simulink model "ddc_bpm_476_066_bak5"  (Simulink 7.8)
settings: Solver=ode45  StartTime=0.0  StopTime=2.56e-3  RelTol=1e-3
undefined symbols (not defined in the file): dt_sim, frev_476, Fs_adc, xlipgetpartsetting
libraries: xbsIndex_r4 x605, simulink x3
(part 2 of 6)

== system ddc_bpm_476_066_bak5/Channel1_fofb ==
  Mix_q_in : Inport
  Mix_i_in : Inport  Port=2
  Analysis : Subsystem
  Goto Tag Visibility3 : GotoTagVisibility  GotoTag=CIC_FOFB_Q_FPGA_OUT
  Goto Tag Visibility4 : GotoTagVisibility  GotoTag=CIC_FOFB_I_FPGA_OUT
  Goto Tag Visibility5 : GotoTagVisibility  GotoTag=CORDIC_FOFB_T_FPGA_OUT
  Goto Tag Visibility6 : GotoTagVisibility  GotoTag=CORDIC_FOFB_R_FPGA_OUT
  Register4 : xbsIndex_r4/Register  init=0  rst=off  en=on  dbl_ovrd=off  block_type=register
  Register5 : xbsIndex_r4/Register  init=0  rst=off  en=on  dbl_ovrd=off  block_type=register
  Register6 : xbsIndex_r4/Register  init=0  rst=off  en=off  dbl_ovrd=off  block_type=register
  Reinterpret2 : xbsIndex_r4/Reinterpret  force_arith_type=off  arith_type=Unsigned  force_bin_pt=off  bin_pt=18  block_type=reinterpret
  Reinterpret3 : xbsIndex_r4/Reinterpret  force_arith_type=off  arith_type=Unsigned  force_bin_pt=off  bin_pt=19  block_type=reinterpret
  Terminator{1,5,8..9} (4 alike) : Terminator
  cic_fofb : Subsystem
  cic_fofb_ch1_i_o : xbsIndex_r4/Gateway Out  inherit_from_input=on  hdl_port=on  timing_constraint=Data Rate  locs_specified=off  LOCs={}  UseAsDAC=off  DACChannel='1'  block_type=gatewayout
      settings: infoedit="Gateway out block.  Converts Xilinx fixed-point or floating-point type inputs into ouputs of type Simulink integer, single, double, or fixed point.<br><br>Hardware notes:  In hardware these blocks become top level output ports or are discarded, depending on how they are configured."
  cic_fofb_ch1_q_o : xbsIndex_r4/Gateway Out  inherit_from_input=on  hdl_port=on  timing_constraint=Data Rate  locs_specified=off  LOCs={}  UseAsDAC=off  DACChannel='1'  block_type=gatewayout
      settings: infoedit="Gateway out block.  Converts Xilinx fixed-point or floating-point type inputs into ouputs of type Simulink integer, single, double, or fixed point.<br><br>Hardware notes:  In hardware these blocks become top level output ports or are discarded, depending on how they are configured."
  fofb_amp_ch1_o : xbsIndex_r4/Gateway Out  inherit_from_input=on  hdl_port=on  timing_constraint=Data Rate  locs_specified=off  LOCs={}  UseAsDAC=off  DACChannel='1'  block_type=gatewayout
      settings: infoedit="Gateway out block.  Converts Xilinx fixed-point or floating-point type inputs into ouputs of type Simulink integer, single, double, or fixed point.<br><br>Hardware notes:  In hardware these blocks become top level output ports or are discarded, depending on how they are configured."
  rect2pol : xbsIndex_r4/CORDIC 5.0   functional_selection=Translate  architectural_configuration=Parallel  pipelining_mode=Maximum  data_format=SignedFraction  phase_format=Radians  input_width=24  output_width=24  round_mode=Nearest_Even  iterations=0  precision=0  compensation_scaling=BRAM  coarse_rotation=on  aclken=off  aresetn=off  out_tready=off  cartesian_has_tuser=off  cartesian_has_tlast=off  cartesian_tuser_width=1  phase_has_tuser=off  phase_has_tlast=off  phase_tuser_width=1  out_tlast_behv=Null  flow_control=NonBlocking  optimize_goal=Resources  trim_axipin_name=on  ip_name=CORDIC  ip_version=5.0  dsptool_ready=true  ipcore_usecache=true  ipcore_useipmodelcache=true  wrapper_available=true  port_translation_map={ 'aclken' => 'en', 'aresetn' => 'rst' }  block_type=cordic_v5_0
      settings: infoedit=CORDIC 5.0
  Amp_F : Outport
  Phase_F : Outport  Port=2
  Valid_F : Outport  Port=3
  tag scope: CIC_FOFB_I_FPGA_OUT=scoped, CIC_FOFB_Q_FPGA_OUT=scoped, CORDIC_FOFB_R_FPGA_OUT=scoped, CORDIC_FOFB_T_FPGA_OUT=scoped
  wires:
  cic_fofb/3(I_out) -> cic_fofb_ch1_i_o/1, [CIC_FOFB_I_FPGA_OUT], rect2pol/3
  cic_fofb/1(Q_out) -> [CIC_FOFB_Q_FPGA_OUT], cic_fofb_ch1_q_o/1, rect2pol/2
  cic_fofb/2(Q_valid) -> Terminator1/1
  rect2pol/1 -> Register4/2, Register5/2, Register6/1
  rect2pol/2 -> Reinterpret2/1
  rect2pol/3 -> Reinterpret3/1
  Register4/1 -> Phase_F/1, [CORDIC_FOFB_T_FPGA_OUT]
  Register5/1 -> Amp_F/1, [CORDIC_FOFB_R_FPGA_OUT], fofb_amp_ch1_o/1
  Register6/1 -> Valid_F/1
  Reinterpret2/1 -> Register4/1
  Reinterpret3/1 -> Register5/1
  fofb_amp_ch1_o/1 -> Terminator5/1
  cic_fofb_ch1_q_o/1 -> Terminator9/1
  cic_fofb_ch1_i_o/1 -> Terminator8/1
  Mix_q_in/1 -> cic_fofb/1(Q_in)
  Mix_i_in/1 -> cic_fofb/2(I_in)
  cic_fofb/4(I_valid) -> rect2pol/1

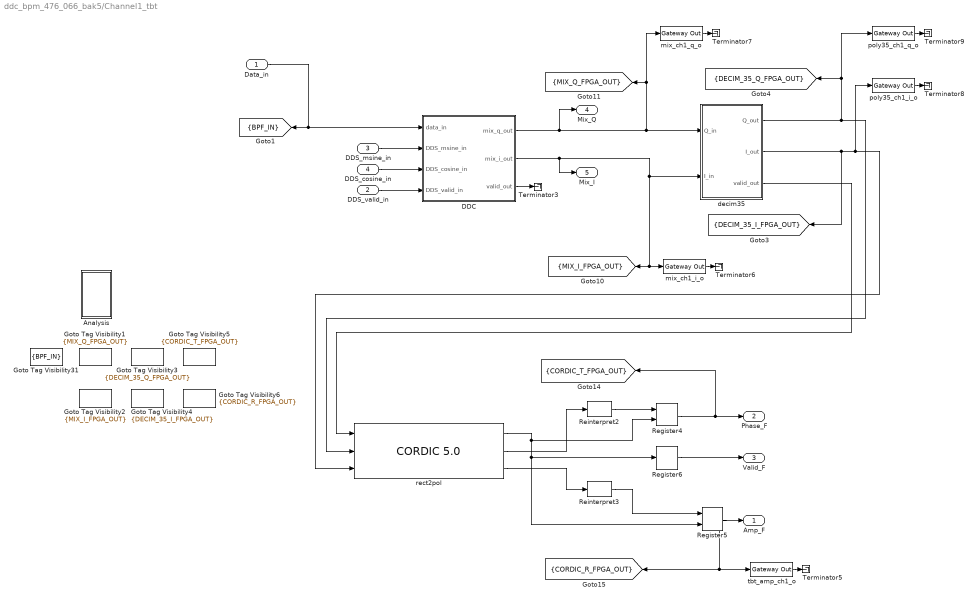
== system ddc_bpm_476_066_bak5/Channel1_tbt ==
  Data_in : Inport
  DDS_valid_in : Inport  Port=2
  DDS_msine_in : Inport  Port=3
  DDS_cosine_in : Inport  Port=4
  Analysis : Subsystem
  DDC : Subsystem
  Goto Tag Visibility1 : GotoTagVisibility  GotoTag=MIX_Q_FPGA_OUT
  Goto Tag Visibility2 : GotoTagVisibility  GotoTag=MIX_I_FPGA_OUT
  Goto Tag Visibility3 : GotoTagVisibility  GotoTag=DECIM_35_Q_FPGA_OUT
  Goto Tag Visibility31 : GotoTagVisibility  GotoTag=BPF_IN
  Goto Tag Visibility4 : GotoTagVisibility  GotoTag=DECIM_35_I_FPGA_OUT
  Goto Tag Visibility5 : GotoTagVisibility  GotoTag=CORDIC_T_FPGA_OUT
  Goto Tag Visibility6 : GotoTagVisibility  GotoTag=CORDIC_R_FPGA_OUT
  Register4 : xbsIndex_r4/Register  init=0  rst=off  en=on  dbl_ovrd=off  block_type=register
  Register5 : xbsIndex_r4/Register  init=0  rst=off  en=on  dbl_ovrd=off  block_type=register
  Register6 : xbsIndex_r4/Register  init=0  rst=off  en=off  dbl_ovrd=off  block_type=register
  Reinterpret2 : xbsIndex_r4/Reinterpret  force_arith_type=off  arith_type=Unsigned  force_bin_pt=off  bin_pt=18  block_type=reinterpret
  Reinterpret3 : xbsIndex_r4/Reinterpret  force_arith_type=off  arith_type=Unsigned  force_bin_pt=off  bin_pt=19  block_type=reinterpret
  Terminator{3,5..9} (6 alike) : Terminator
  decim35 : Subsystem
  mix_ch1_i_o : xbsIndex_r4/Gateway Out  inherit_from_input=on  hdl_port=on  timing_constraint=Data Rate  locs_specified=off  LOCs={}  UseAsDAC=off  DACChannel='1'  block_type=gatewayout
      settings: infoedit="Gateway out block.  Converts Xilinx fixed-point or floating-point type inputs into ouputs of type Simulink integer, single, double, or fixed point.<br><br>Hardware notes:  In hardware these blocks become top level output ports or are discarded, depending on how they are configured."
  mix_ch1_q_o : xbsIndex_r4/Gateway Out  inherit_from_input=on  hdl_port=on  timing_constraint=Data Rate  locs_specified=off  LOCs={}  UseAsDAC=off  DACChannel='1'  block_type=gatewayout
      settings: infoedit="Gateway out block.  Converts Xilinx fixed-point or floating-point type inputs into ouputs of type Simulink integer, single, double, or fixed point.<br><br>Hardware notes:  In hardware these blocks become top level output ports or are discarded, depending on how they are configured."
  poly35_ch1_i_o : xbsIndex_r4/Gateway Out  inherit_from_input=on  hdl_port=on  timing_constraint=Data Rate  locs_specified=off  LOCs={}  UseAsDAC=off  DACChannel='1'  block_type=gatewayout
      settings: infoedit="Gateway out block.  Converts Xilinx fixed-point or floating-point type inputs into ouputs of type Simulink integer, single, double, or fixed point.<br><br>Hardware notes:  In hardware these blocks become top level output ports or are discarded, depending on how they are configured."
  poly35_ch1_q_o : xbsIndex_r4/Gateway Out  inherit_from_input=on  hdl_port=on  timing_constraint=Data Rate  locs_specified=off  LOCs={}  UseAsDAC=off  DACChannel='1'  block_type=gatewayout
      settings: infoedit="Gateway out block.  Converts Xilinx fixed-point or floating-point type inputs into ouputs of type Simulink integer, single, double, or fixed point.<br><br>Hardware notes:  In hardware these blocks become top level output ports or are discarded, depending on how they are configured."
  rect2pol : xbsIndex_r4/CORDIC 5.0   functional_selection=Translate  architectural_configuration=Parallel  pipelining_mode=Maximum  data_format=SignedFraction  phase_format=Radians  input_width=24  output_width=24  round_mode=Nearest_Even  iterations=0  precision=0  compensation_scaling=BRAM  coarse_rotation=on  aclken=off  aresetn=off  out_tready=off  cartesian_has_tuser=off  cartesian_has_tlast=off  cartesian_tuser_width=1  phase_has_tuser=off  phase_has_tlast=off  phase_tuser_width=1  out_tlast_behv=Null  flow_control=NonBlocking  optimize_goal=Resources  trim_axipin_name=on  ip_name=CORDIC  ip_version=5.0  dsptool_ready=true  ipcore_usecache=true  ipcore_useipmodelcache=true  wrapper_available=true  port_translation_map={ 'aclken' => 'en', 'aresetn' => 'rst' }  block_type=cordic_v5_0
      settings: infoedit=CORDIC 5.0
  tbt_amp_ch1_o : xbsIndex_r4/Gateway Out  inherit_from_input=on  hdl_port=on  timing_constraint=Data Rate  locs_specified=off  LOCs={}  UseAsDAC=off  DACChannel='1'  block_type=gatewayout
      settings: infoedit="Gateway out block.  Converts Xilinx fixed-point or floating-point type inputs into ouputs of type Simulink integer, single, double, or fixed point.<br><br>Hardware notes:  In hardware these blocks become top level output ports or are discarded, depending on how they are configured."
  Amp_F : Outport
  Phase_F : Outport  Port=2
  Valid_F : Outport  Port=3
  Mix_Q : Outport  Port=4
  Mix_I : Outport  Port=5
  tag scope: BPF_IN=scoped, CORDIC_R_FPGA_OUT=scoped, CORDIC_T_FPGA_OUT=scoped, DECIM_35_I_FPGA_OUT=scoped, DECIM_35_Q_FPGA_OUT=scoped, MIX_I_FPGA_OUT=scoped, MIX_Q_FPGA_OUT=scoped
  wires:
  Data_in/1 -> [BPF_IN], DDC/1(data_in)
  DDC/2(mix_i_out) -> [MIX_I_FPGA_OUT], mix_ch1_i_o/1, decim35/2(I_in), Mix_I/1
  DDC/3(valid_out) -> Terminator3/1
  DDC/1(mix_q_out) -> [MIX_Q_FPGA_OUT], mix_ch1_q_o/1, decim35/1(Q_in), Mix_Q/1
  decim35/2(I_out) -> [DECIM_35_I_FPGA_OUT], poly35_ch1_i_o/1, rect2pol/3
  decim35/1(Q_out) -> [DECIM_35_Q_FPGA_OUT], poly35_ch1_q_o/1, rect2pol/2
  decim35/3(valid_out) -> rect2pol/1
  rect2pol/1 -> Register4/2, Register5/2, Register6/1
  rect2pol/2 -> Reinterpret2/1
  rect2pol/3 -> Reinterpret3/1
  Register4/1 -> Phase_F/1, [CORDIC_T_FPGA_OUT]
  Register5/1 -> Amp_F/1, [CORDIC_R_FPGA_OUT], tbt_amp_ch1_o/1
  Register6/1 -> Valid_F/1
  Reinterpret2/1 -> Register4/1
  Reinterpret3/1 -> Register5/1
  tbt_amp_ch1_o/1 -> Terminator5/1
  mix_ch1_i_o/1 -> Terminator6/1
  mix_ch1_q_o/1 -> Terminator7/1
  poly35_ch1_q_o/1 -> Terminator9/1
  poly35_ch1_i_o/1 -> Terminator8/1
  DDS_valid_in/1 -> DDC/4(DDS_valid_in)
  DDS_msine_in/1 -> DDC/2(DDS_msine_in)
  DDS_cosine_in/1 -> DDC/3(DDS_cosine_in)

== system ddc_bpm_476_066_bak5/Channel2_fofb ==
  Mix_q_in : Inport
  Mix_i_in : Inport  Port=2
  Analysis : Subsystem
  Goto Tag Visibility3 : GotoTagVisibility  GotoTag=CIC_FOFB_Q_FPGA_OUT
  Goto Tag Visibility4 : GotoTagVisibility  GotoTag=CIC_FOFB_I_FPGA_OUT
  Goto Tag Visibility5 : GotoTagVisibility  GotoTag=CORDIC_FOFB_T_FPGA_OUT
  Goto Tag Visibility6 : GotoTagVisibility  GotoTag=CORDIC_FOFB_R_FPGA_OUT
  Register4 : xbsIndex_r4/Register  init=0  rst=off  en=on  dbl_ovrd=off  block_type=register
  Register5 : xbsIndex_r4/Register  init=0  rst=off  en=on  dbl_ovrd=off  block_type=register
  Register6 : xbsIndex_r4/Register  init=0  rst=off  en=off  dbl_ovrd=off  block_type=register
  Reinterpret2 : xbsIndex_r4/Reinterpret  force_arith_type=off  arith_type=Unsigned  force_bin_pt=off  bin_pt=18  block_type=reinterpret
  Reinterpret3 : xbsIndex_r4/Reinterpret  force_arith_type=off  arith_type=Unsigned  force_bin_pt=off  bin_pt=19  block_type=reinterpret
  Terminator{1,5,8..9} (4 alike) : Terminator
  cic_fofb : Subsystem
  cic_fofb_ch2_i_o : xbsIndex_r4/Gateway Out  inherit_from_input=on  hdl_port=on  timing_constraint=Data Rate  locs_specified=off  LOCs={}  UseAsDAC=off  DACChannel='1'  block_type=gatewayout
      settings: infoedit="Gateway out block.  Converts Xilinx fixed-point or floating-point type inputs into ouputs of type Simulink integer, single, double, or fixed point.<br><br>Hardware notes:  In hardware these blocks become top level output ports or are discarded, depending on how they are configured."
  cic_fofb_ch2_q_o : xbsIndex_r4/Gateway Out  inherit_from_input=on  hdl_port=on  timing_constraint=Data Rate  locs_specified=off  LOCs={}  UseAsDAC=off  DACChannel='1'  block_type=gatewayout
      settings: infoedit="Gateway out block.  Converts Xilinx fixed-point or floating-point type inputs into ouputs of type Simulink integer, single, double, or fixed point.<br><br>Hardware notes:  In hardware these blocks become top level output ports or are discarded, depending on how they are configured."
  fofb_amp_ch2_o : xbsIndex_r4/Gateway Out  inherit_from_input=on  hdl_port=on  timing_constraint=Data Rate  locs_specified=off  LOCs={}  UseAsDAC=off  DACChannel='1'  block_type=gatewayout
      settings: infoedit="Gateway out block.  Converts Xilinx fixed-point or floating-point type inputs into ouputs of type Simulink integer, single, double, or fixed point.<br><br>Hardware notes:  In hardware these blocks become top level output ports or are discarded, depending on how they are configured."
  rect2pol : xbsIndex_r4/CORDIC 5.0   functional_selection=Translate  architectural_configuration=Parallel  pipelining_mode=Maximum  data_format=SignedFraction  phase_format=Radians  input_width=24  output_width=24  round_mode=Nearest_Even  iterations=0  precision=0  compensation_scaling=BRAM  coarse_rotation=on  aclken=off  aresetn=off  out_tready=off  cartesian_has_tuser=off  cartesian_has_tlast=off  cartesian_tuser_width=1  phase_has_tuser=off  phase_has_tlast=off  phase_tuser_width=1  out_tlast_behv=Null  flow_control=NonBlocking  optimize_goal=Resources  trim_axipin_name=on  ip_name=CORDIC  ip_version=5.0  dsptool_ready=true  ipcore_usecache=true  ipcore_useipmodelcache=true  wrapper_available=true  port_translation_map={ 'aclken' => 'en', 'aresetn' => 'rst' }  block_type=cordic_v5_0
      settings: infoedit=CORDIC 5.0
  Amp_F : Outport
  Phase_F : Outport  Port=2
  Valid_F : Outport  Port=3
  tag scope: CIC_FOFB_I_FPGA_OUT=scoped, CIC_FOFB_Q_FPGA_OUT=scoped, CORDIC_FOFB_R_FPGA_OUT=scoped, CORDIC_FOFB_T_FPGA_OUT=scoped
  wires:
  cic_fofb/3(I_out) -> cic_fofb_ch2_i_o/1, [CIC_FOFB_I_FPGA_OUT], rect2pol/3
  cic_fofb/1(Q_out) -> [CIC_FOFB_Q_FPGA_OUT], cic_fofb_ch2_q_o/1, rect2pol/2
  cic_fofb/2(Q_valid) -> Terminator1/1
  rect2pol/1 -> Register4/2, Register5/2, Register6/1
  rect2pol/2 -> Reinterpret2/1
  rect2pol/3 -> Reinterpret3/1
  Register4/1 -> Phase_F/1, [CORDIC_FOFB_T_FPGA_OUT]
  Register5/1 -> Amp_F/1, [CORDIC_FOFB_R_FPGA_OUT], fofb_amp_ch2_o/1
  Register6/1 -> Valid_F/1
  Reinterpret2/1 -> Register4/1
  Reinterpret3/1 -> Register5/1
  fofb_amp_ch2_o/1 -> Terminator5/1
  cic_fofb_ch2_q_o/1 -> Terminator9/1
  cic_fofb_ch2_i_o/1 -> Terminator8/1
  Mix_q_in/1 -> cic_fofb/1(Q_in)
  Mix_i_in/1 -> cic_fofb/2(I_in)
  cic_fofb/4(I_valid) -> rect2pol/1

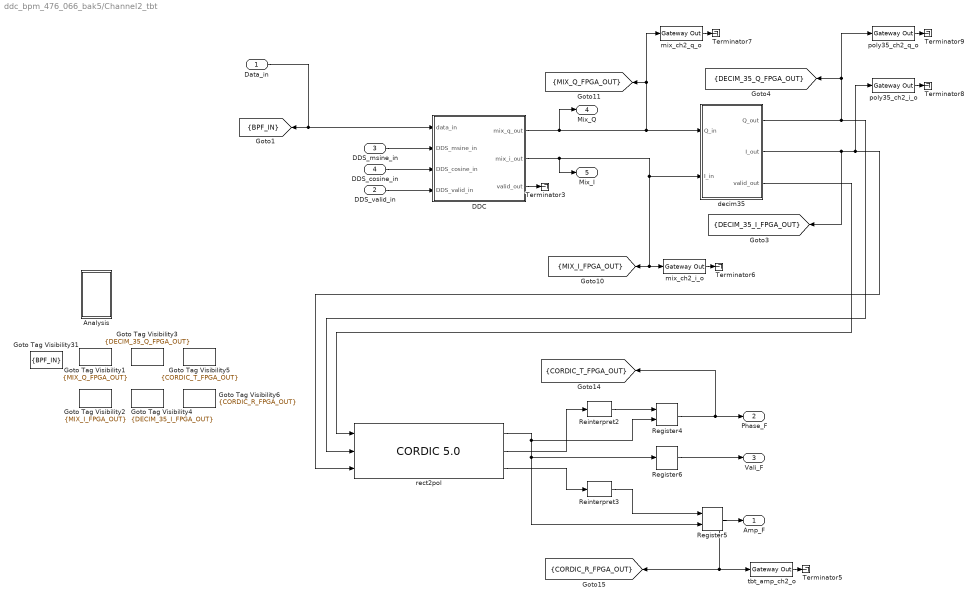
== system ddc_bpm_476_066_bak5/Channel2_tbt ==
  Data_in : Inport
  DDS_valid_in : Inport  Port=2
  DDS_msine_in : Inport  Port=3
  DDS_cosine_in : Inport  Port=4
  Analysis : Subsystem
  DDC : Subsystem
  Goto Tag Visibility1 : GotoTagVisibility  GotoTag=MIX_Q_FPGA_OUT
  Goto Tag Visibility2 : GotoTagVisibility  GotoTag=MIX_I_FPGA_OUT
  Goto Tag Visibility3 : GotoTagVisibility  GotoTag=DECIM_35_Q_FPGA_OUT
  Goto Tag Visibility31 : GotoTagVisibility  GotoTag=BPF_IN
  Goto Tag Visibility4 : GotoTagVisibility  GotoTag=DECIM_35_I_FPGA_OUT
  Goto Tag Visibility5 : GotoTagVisibility  GotoTag=CORDIC_T_FPGA_OUT
  Goto Tag Visibility6 : GotoTagVisibility  GotoTag=CORDIC_R_FPGA_OUT
  Register4 : xbsIndex_r4/Register  init=0  rst=off  en=on  dbl_ovrd=off  block_type=register
  Register5 : xbsIndex_r4/Register  init=0  rst=off  en=on  dbl_ovrd=off  block_type=register
  Register6 : xbsIndex_r4/Register  init=0  rst=off  en=off  dbl_ovrd=off  block_type=register
  Reinterpret2 : xbsIndex_r4/Reinterpret  force_arith_type=off  arith_type=Unsigned  force_bin_pt=off  bin_pt=18  block_type=reinterpret
  Reinterpret3 : xbsIndex_r4/Reinterpret  force_arith_type=off  arith_type=Unsigned  force_bin_pt=off  bin_pt=19  block_type=reinterpret
  Terminator{3,5..9} (6 alike) : Terminator
  decim35 : Subsystem
  mix_ch2_i_o : xbsIndex_r4/Gateway Out  inherit_from_input=on  hdl_port=on  timing_constraint=Data Rate  locs_specified=off  LOCs={}  UseAsDAC=off  DACChannel='1'  block_type=gatewayout
      settings: infoedit="Gateway out block.  Converts Xilinx fixed-point or floating-point type inputs into ouputs of type Simulink integer, single, double, or fixed point.<br><br>Hardware notes:  In hardware these blocks become top level output ports or are discarded, depending on how they are configured."
  mix_ch2_q_o : xbsIndex_r4/Gateway Out  inherit_from_input=on  hdl_port=on  timing_constraint=Data Rate  locs_specified=off  LOCs={}  UseAsDAC=off  DACChannel='1'  block_type=gatewayout
      settings: infoedit="Gateway out block.  Converts Xilinx fixed-point or floating-point type inputs into ouputs of type Simulink integer, single, double, or fixed point.<br><br>Hardware notes:  In hardware these blocks become top level output ports or are discarded, depending on how they are configured."
  poly35_ch2_i_o : xbsIndex_r4/Gateway Out  inherit_from_input=on  hdl_port=on  timing_constraint=Data Rate  locs_specified=off  LOCs={}  UseAsDAC=off  DACChannel='1'  block_type=gatewayout
      settings: infoedit="Gateway out block.  Converts Xilinx fixed-point or floating-point type inputs into ouputs of type Simulink integer, single, double, or fixed point.<br><br>Hardware notes:  In hardware these blocks become top level output ports or are discarded, depending on how they are configured."
  poly35_ch2_q_o : xbsIndex_r4/Gateway Out  inherit_from_input=on  hdl_port=on  timing_constraint=Data Rate  locs_specified=off  LOCs={}  UseAsDAC=off  DACChannel='1'  block_type=gatewayout
      settings: infoedit="Gateway out block.  Converts Xilinx fixed-point or floating-point type inputs into ouputs of type Simulink integer, single, double, or fixed point.<br><br>Hardware notes:  In hardware these blocks become top level output ports or are discarded, depending on how they are configured."
  rect2pol : xbsIndex_r4/CORDIC 5.0   functional_selection=Translate  architectural_configuration=Parallel  pipelining_mode=Maximum  data_format=SignedFraction  phase_format=Radians  input_width=24  output_width=24  round_mode=Nearest_Even  iterations=0  precision=0  compensation_scaling=BRAM  coarse_rotation=on  aclken=off  aresetn=off  out_tready=off  cartesian_has_tuser=off  cartesian_has_tlast=off  cartesian_tuser_width=1  phase_has_tuser=off  phase_has_tlast=off  phase_tuser_width=1  out_tlast_behv=Null  flow_control=NonBlocking  optimize_goal=Resources  trim_axipin_name=on  ip_name=CORDIC  ip_version=5.0  dsptool_ready=true  ipcore_usecache=true  ipcore_useipmodelcache=true  wrapper_available=true  port_translation_map={ 'aclken' => 'en', 'aresetn' => 'rst' }  block_type=cordic_v5_0
      settings: infoedit=CORDIC 5.0
  tbt_amp_ch2_o : xbsIndex_r4/Gateway Out  inherit_from_input=on  hdl_port=on  timing_constraint=Data Rate  locs_specified=off  LOCs={}  UseAsDAC=off  DACChannel='1'  block_type=gatewayout
      settings: infoedit="Gateway out block.  Converts Xilinx fixed-point or floating-point type inputs into ouputs of type Simulink integer, single, double, or fixed point.<br><br>Hardware notes:  In hardware these blocks become top level output ports or are discarded, depending on how they are configured."
  Amp_F : Outport
  Phase_F : Outport  Port=2
  Vali_F : Outport  Port=3
  Mix_Q : Outport  Port=4
  Mix_I : Outport  Port=5
  tag scope: BPF_IN=scoped, CORDIC_R_FPGA_OUT=scoped, CORDIC_T_FPGA_OUT=scoped, DECIM_35_I_FPGA_OUT=scoped, DECIM_35_Q_FPGA_OUT=scoped, MIX_I_FPGA_OUT=scoped, MIX_Q_FPGA_OUT=scoped
  wires:
  Data_in/1 -> [BPF_IN], DDC/1(data_in)
  DDC/2(mix_i_out) -> [MIX_I_FPGA_OUT], mix_ch2_i_o/1, decim35/2(I_in), Mix_I/1
  DDC/3(valid_out) -> Terminator3/1
  DDC/1(mix_q_out) -> [MIX_Q_FPGA_OUT], mix_ch2_q_o/1, decim35/1(Q_in), Mix_Q/1
  decim35/2(I_out) -> [DECIM_35_I_FPGA_OUT], poly35_ch2_i_o/1, rect2pol/3
  decim35/1(Q_out) -> [DECIM_35_Q_FPGA_OUT], poly35_ch2_q_o/1, rect2pol/2
  decim35/3(valid_out) -> rect2pol/1
  rect2pol/1 -> Register4/2, Register5/2, Register6/1
  rect2pol/2 -> Reinterpret2/1
  rect2pol/3 -> Reinterpret3/1
  Register4/1 -> Phase_F/1, [CORDIC_T_FPGA_OUT]
  Register5/1 -> Amp_F/1, [CORDIC_R_FPGA_OUT], tbt_amp_ch2_o/1
  Register6/1 -> Vali_F/1
  Reinterpret2/1 -> Register4/1
  Reinterpret3/1 -> Register5/1
  tbt_amp_ch2_o/1 -> Terminator5/1
  mix_ch2_i_o/1 -> Terminator6/1
  mix_ch2_q_o/1 -> Terminator7/1
  poly35_ch2_q_o/1 -> Terminator9/1
  poly35_ch2_i_o/1 -> Terminator8/1
  DDS_valid_in/1 -> DDC/4(DDS_valid_in)
  DDS_msine_in/1 -> DDC/2(DDS_msine_in)
  DDS_cosine_in/1 -> DDC/3(DDS_cosine_in)

== system ddc_bpm_476_066_bak5/Channel3_fofb ==
  Mix_q_in : Inport
  Mix_i_in : Inport  Port=2
  Analysis : Subsystem
  Goto Tag Visibility3 : GotoTagVisibility  GotoTag=CIC_FOFB_Q_FPGA_OUT
  Goto Tag Visibility4 : GotoTagVisibility  GotoTag=CIC_FOFB_I_FPGA_OUT
  Goto Tag Visibility5 : GotoTagVisibility  GotoTag=CORDIC_FOFB_T_FPGA_OUT
  Goto Tag Visibility6 : GotoTagVisibility  GotoTag=CORDIC_FOFB_R_FPGA_OUT
  Register4 : xbsIndex_r4/Register  init=0  rst=off  en=on  dbl_ovrd=off  block_type=register
  Register5 : xbsIndex_r4/Register  init=0  rst=off  en=on  dbl_ovrd=off  block_type=register
  Register6 : xbsIndex_r4/Register  init=0  rst=off  en=off  dbl_ovrd=off  block_type=register
  Reinterpret2 : xbsIndex_r4/Reinterpret  force_arith_type=off  arith_type=Unsigned  force_bin_pt=off  bin_pt=18  block_type=reinterpret
  Reinterpret3 : xbsIndex_r4/Reinterpret  force_arith_type=off  arith_type=Unsigned  force_bin_pt=off  bin_pt=19  block_type=reinterpret
  Terminator{1,5,8..9} (4 alike) : Terminator
  cic_fofb : Subsystem
  cic_fofb_ch3_i_o : xbsIndex_r4/Gateway Out  inherit_from_input=on  hdl_port=on  timing_constraint=Data Rate  locs_specified=off  LOCs={}  UseAsDAC=off  DACChannel='1'  block_type=gatewayout
      settings: infoedit="Gateway out block.  Converts Xilinx fixed-point or floating-point type inputs into ouputs of type Simulink integer, single, double, or fixed point.<br><br>Hardware notes:  In hardware these blocks become top level output ports or are discarded, depending on how they are configured."
  cic_fofb_ch3_q_o : xbsIndex_r4/Gateway Out  inherit_from_input=on  hdl_port=on  timing_constraint=Data Rate  locs_specified=off  LOCs={}  UseAsDAC=off  DACChannel='1'  block_type=gatewayout
      settings: infoedit="Gateway out block.  Converts Xilinx fixed-point or floating-point type inputs into ouputs of type Simulink integer, single, double, or fixed point.<br><br>Hardware notes:  In hardware these blocks become top level output ports or are discarded, depending on how they are configured."
  fofb_amp_ch3_o : xbsIndex_r4/Gateway Out  inherit_from_input=on  hdl_port=on  timing_constraint=Data Rate  locs_specified=off  LOCs={}  UseAsDAC=off  DACChannel='1'  block_type=gatewayout
      settings: infoedit="Gateway out block.  Converts Xilinx fixed-point or floating-point type inputs into ouputs of type Simulink integer, single, double, or fixed point.<br><br>Hardware notes:  In hardware these blocks become top level output ports or are discarded, depending on how they are configured."
  rect2pol : xbsIndex_r4/CORDIC 5.0   functional_selection=Translate  architectural_configuration=Parallel  pipelining_mode=Maximum  data_format=SignedFraction  phase_format=Radians  input_width=24  output_width=24  round_mode=Nearest_Even  iterations=0  precision=0  compensation_scaling=BRAM  coarse_rotation=on  aclken=off  aresetn=off  out_tready=off  cartesian_has_tuser=off  cartesian_has_tlast=off  cartesian_tuser_width=1  phase_has_tuser=off  phase_has_tlast=off  phase_tuser_width=1  out_tlast_behv=Null  flow_control=NonBlocking  optimize_goal=Resources  trim_axipin_name=on  ip_name=CORDIC  ip_version=5.0  dsptool_ready=true  ipcore_usecache=true  ipcore_useipmodelcache=true  wrapper_available=true  port_translation_map={ 'aclken' => 'en', 'aresetn' => 'rst' }  block_type=cordic_v5_0
      settings: infoedit=CORDIC 5.0
  Amp_F : Outport
  Phase_F : Outport  Port=2
  Valid_F : Outport  Port=3
  tag scope: CIC_FOFB_I_FPGA_OUT=scoped, CIC_FOFB_Q_FPGA_OUT=scoped, CORDIC_FOFB_R_FPGA_OUT=scoped, CORDIC_FOFB_T_FPGA_OUT=scoped
  wires:
  cic_fofb/3(I_out) -> cic_fofb_ch3_i_o/1, [CIC_FOFB_I_FPGA_OUT], rect2pol/3
  cic_fofb/1(Q_out) -> [CIC_FOFB_Q_FPGA_OUT], cic_fofb_ch3_q_o/1, rect2pol/2
  cic_fofb/2(Q_valid) -> Terminator1/1
  rect2pol/1 -> Register4/2, Register5/2, Register6/1
  rect2pol/2 -> Reinterpret2/1
  rect2pol/3 -> Reinterpret3/1
  Register4/1 -> Phase_F/1, [CORDIC_FOFB_T_FPGA_OUT]
  Register5/1 -> Amp_F/1, [CORDIC_FOFB_R_FPGA_OUT], fofb_amp_ch3_o/1
  Register6/1 -> Valid_F/1
  Reinterpret2/1 -> Register4/1
  Reinterpret3/1 -> Register5/1
  fofb_amp_ch3_o/1 -> Terminator5/1
  cic_fofb_ch3_q_o/1 -> Terminator9/1
  cic_fofb_ch3_i_o/1 -> Terminator8/1
  Mix_q_in/1 -> cic_fofb/1(Q_in)
  Mix_i_in/1 -> cic_fofb/2(I_in)
  cic_fofb/4(I_valid) -> rect2pol/1

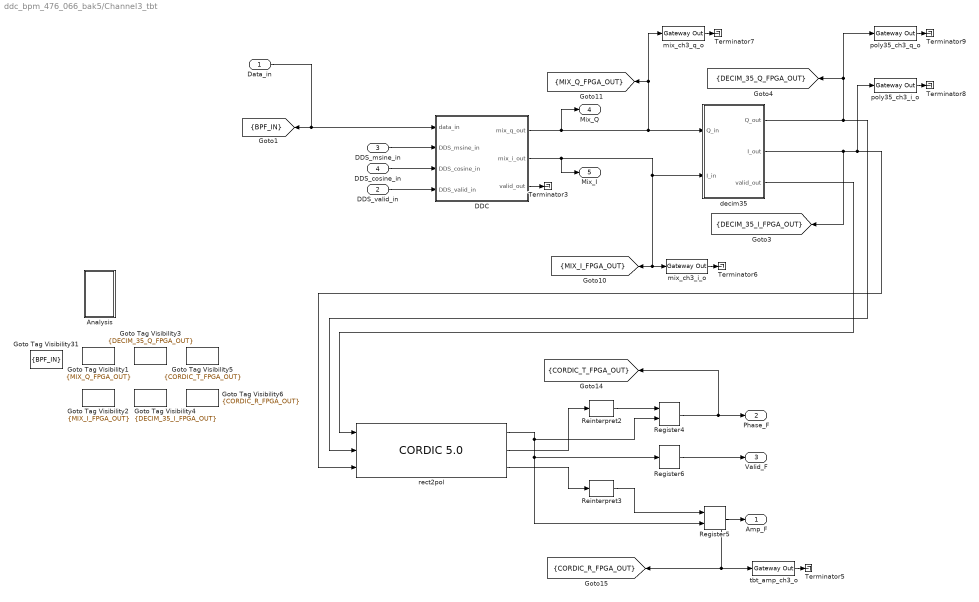
== system ddc_bpm_476_066_bak5/Channel3_tbt ==
  Data_in : Inport
  DDS_valid_in : Inport  Port=2
  DDS_msine_in : Inport  Port=3
  DDS_cosine_in : Inport  Port=4
  Analysis : Subsystem
  DDC : Subsystem
  Goto Tag Visibility1 : GotoTagVisibility  GotoTag=MIX_Q_FPGA_OUT
  Goto Tag Visibility2 : GotoTagVisibility  GotoTag=MIX_I_FPGA_OUT
  Goto Tag Visibility3 : GotoTagVisibility  GotoTag=DECIM_35_Q_FPGA_OUT
  Goto Tag Visibility31 : GotoTagVisibility  GotoTag=BPF_IN
  Goto Tag Visibility4 : GotoTagVisibility  GotoTag=DECIM_35_I_FPGA_OUT
  Goto Tag Visibility5 : GotoTagVisibility  GotoTag=CORDIC_T_FPGA_OUT
  Goto Tag Visibility6 : GotoTagVisibility  GotoTag=CORDIC_R_FPGA_OUT
  Register4 : xbsIndex_r4/Register  init=0  rst=off  en=on  dbl_ovrd=off  block_type=register
  Register5 : xbsIndex_r4/Register  init=0  rst=off  en=on  dbl_ovrd=off  block_type=register
  Register6 : xbsIndex_r4/Register  init=0  rst=off  en=off  dbl_ovrd=off  block_type=register
  Reinterpret2 : xbsIndex_r4/Reinterpret  force_arith_type=off  arith_type=Unsigned  force_bin_pt=off  bin_pt=18  block_type=reinterpret
  Reinterpret3 : xbsIndex_r4/Reinterpret  force_arith_type=off  arith_type=Unsigned  force_bin_pt=off  bin_pt=19  block_type=reinterpret
  Terminator{3,5..9} (6 alike) : Terminator
  decim35 : Subsystem
  mix_ch3_i_o : xbsIndex_r4/Gateway Out  inherit_from_input=on  hdl_port=on  timing_constraint=Data Rate  locs_specified=off  LOCs={}  UseAsDAC=off  DACChannel='1'  block_type=gatewayout
      settings: infoedit="Gateway out block.  Converts Xilinx fixed-point or floating-point type inputs into ouputs of type Simulink integer, single, double, or fixed point.<br><br>Hardware notes:  In hardware these blocks become top level output ports or are discarded, depending on how they are configured."
  mix_ch3_q_o : xbsIndex_r4/Gateway Out  inherit_from_input=on  hdl_port=on  timing_constraint=Data Rate  locs_specified=off  LOCs={}  UseAsDAC=off  DACChannel='1'  block_type=gatewayout
      settings: infoedit="Gateway out block.  Converts Xilinx fixed-point or floating-point type inputs into ouputs of type Simulink integer, single, double, or fixed point.<br><br>Hardware notes:  In hardware these blocks become top level output ports or are discarded, depending on how they are configured."
  poly35_ch3_i_o : xbsIndex_r4/Gateway Out  inherit_from_input=on  hdl_port=on  timing_constraint=Data Rate  locs_specified=off  LOCs={}  UseAsDAC=off  DACChannel='1'  block_type=gatewayout
      settings: infoedit="Gateway out block.  Converts Xilinx fixed-point or floating-point type inputs into ouputs of type Simulink integer, single, double, or fixed point.<br><br>Hardware notes:  In hardware these blocks become top level output ports or are discarded, depending on how they are configured."
  poly35_ch3_q_o : xbsIndex_r4/Gateway Out  inherit_from_input=on  hdl_port=on  timing_constraint=Data Rate  locs_specified=off  LOCs={}  UseAsDAC=off  DACChannel='1'  block_type=gatewayout
      settings: infoedit="Gateway out block.  Converts Xilinx fixed-point or floating-point type inputs into ouputs of type Simulink integer, single, double, or fixed point.<br><br>Hardware notes:  In hardware these blocks become top level output ports or are discarded, depending on how they are configured."
  rect2pol : xbsIndex_r4/CORDIC 5.0   functional_selection=Translate  architectural_configuration=Parallel  pipelining_mode=Maximum  data_format=SignedFraction  phase_format=Radians  input_width=24  output_width=24  round_mode=Nearest_Even  iterations=0  precision=0  compensation_scaling=BRAM  coarse_rotation=on  aclken=off  aresetn=off  out_tready=off  cartesian_has_tuser=off  cartesian_has_tlast=off  cartesian_tuser_width=1  phase_has_tuser=off  phase_has_tlast=off  phase_tuser_width=1  out_tlast_behv=Null  flow_control=NonBlocking  optimize_goal=Resources  trim_axipin_name=on  ip_name=CORDIC  ip_version=5.0  dsptool_ready=true  ipcore_usecache=true  ipcore_useipmodelcache=true  wrapper_available=true  port_translation_map={ 'aclken' => 'en', 'aresetn' => 'rst' }  block_type=cordic_v5_0
      settings: infoedit=CORDIC 5.0
  tbt_amp_ch3_o : xbsIndex_r4/Gateway Out  inherit_from_input=on  hdl_port=on  timing_constraint=Data Rate  locs_specified=off  LOCs={}  UseAsDAC=off  DACChannel='1'  block_type=gatewayout
      settings: infoedit="Gateway out block.  Converts Xilinx fixed-point or floating-point type inputs into ouputs of type Simulink integer, single, double, or fixed point.<br><br>Hardware notes:  In hardware these blocks become top level output ports or are discarded, depending on how they are configured."
  Amp_F : Outport
  Phase_F : Outport  Port=2
  Valid_F : Outport  Port=3
  Mix_Q : Outport  Port=4
  Mix_I : Outport  Port=5
  tag scope: BPF_IN=scoped, CORDIC_R_FPGA_OUT=scoped, CORDIC_T_FPGA_OUT=scoped, DECIM_35_I_FPGA_OUT=scoped, DECIM_35_Q_FPGA_OUT=scoped, MIX_I_FPGA_OUT=scoped, MIX_Q_FPGA_OUT=scoped
  wires:
  Data_in/1 -> [BPF_IN], DDC/1(data_in)
  DDC/2(mix_i_out) -> [MIX_I_FPGA_OUT], mix_ch3_i_o/1, decim35/2(I_in), Mix_I/1
  DDC/3(valid_out) -> Terminator3/1
  DDC/1(mix_q_out) -> [MIX_Q_FPGA_OUT], mix_ch3_q_o/1, decim35/1(Q_in), Mix_Q/1
  decim35/2(I_out) -> [DECIM_35_I_FPGA_OUT], poly35_ch3_i_o/1, rect2pol/3
  decim35/1(Q_out) -> [DECIM_35_Q_FPGA_OUT], poly35_ch3_q_o/1, rect2pol/2
  decim35/3(valid_out) -> rect2pol/1
  rect2pol/1 -> Register4/2, Register5/2, Register6/1
  rect2pol/2 -> Reinterpret2/1
  rect2pol/3 -> Reinterpret3/1
  Register4/1 -> Phase_F/1, [CORDIC_T_FPGA_OUT]
  Register5/1 -> Amp_F/1, [CORDIC_R_FPGA_OUT], tbt_amp_ch3_o/1
  Register6/1 -> Valid_F/1
  Reinterpret2/1 -> Register4/1
  Reinterpret3/1 -> Register5/1
  tbt_amp_ch3_o/1 -> Terminator5/1
  mix_ch3_i_o/1 -> Terminator6/1
  mix_ch3_q_o/1 -> Terminator7/1
  poly35_ch3_q_o/1 -> Terminator9/1
  poly35_ch3_i_o/1 -> Terminator8/1
  DDS_valid_in/1 -> DDC/4(DDS_valid_in)
  DDS_msine_in/1 -> DDC/2(DDS_msine_in)
  DDS_cosine_in/1 -> DDC/3(DDS_cosine_in)
